simulink model "ASE_370C_MinProj2_simulink"  (R2018b)
settings: Solver=VariableStepAuto  StartTime=0.0  StopTime=20  RelTol=1e-3
InitFcn:
  | RUN_1st_ASE_370C_MiniProject1
CloseFcn:
  | ASE_370C_MiniProject1_Plots
settings Model: Creator=kenda  LastModifiedBy=kenda

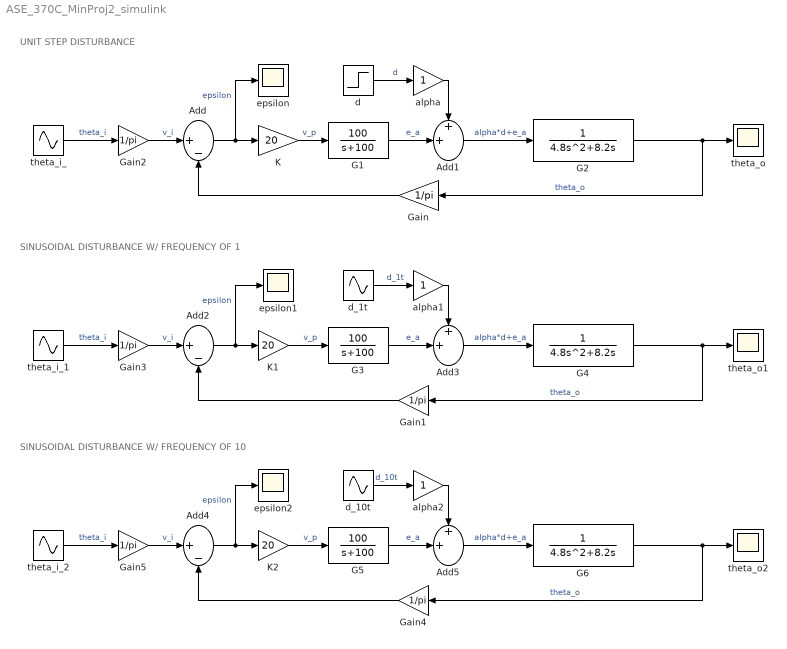
== system ASE_370C_MinProj2_simulink ==
  note: UNIT STEP DISTURBANCE
  note: SINUSOIDAL DISTURBANCE W/ FREQUENCY OF 1
  note: SINUSOIDAL DISTURBANCE W/ FREQUENCY OF 10
  Add : Sum  Inputs=|+-
  Add1 : Sum  Inputs=++|
  Add2 : Sum  Inputs=|+-
  Add3 : Sum  Inputs=++|
  Add4 : Sum  Inputs=|+-
  Add5 : Sum  Inputs=++|
  G1 : TransferFcn  Numerator=100  Denominator=[1 100]
  G2 : TransferFcn  Denominator=[4.8 8.2 0]
  G3 : TransferFcn  Numerator=100  Denominator=[1 100]
  G4 : TransferFcn  Denominator=[4.8 8.2 0]
  G5 : TransferFcn  Numerator=100  Denominator=[1 100]
  G6 : TransferFcn  Denominator=[4.8 8.2 0]
  Gain{,1..5} (6 alike) : Gain  Gain=1/pi
  K : Gain  Gain=20
  K1 : Gain  Gain=20
  K2 : Gain  Gain=20
  alpha : Gain
  alpha1 : Gain
  alpha2 : Gain
  d : Step  SampleTime=0
  d_10t : Sin  Frequency=10  SampleTime=0
  d_1t : Sin  SampleTime=0
  epsilon : Scope
  epsilon1 : Scope
  epsilon2 : Scope
  theta_i_ : Sin  Bias=1  Frequency=0  SampleTime=0
  theta_i_1 : Sin  Frequency=0  SampleTime=0
  theta_i_2 : Sin  Frequency=0  SampleTime=0
  theta_o : Scope
  theta_o1 : Scope
  theta_o2 : Scope
  wires:
  Gain2/1 -> Add/1  "v_i"
  Add/1 -> epsilon/1, K/1  "epsilon"
  K/1 -> G1/1  "v_p"
  G1/1 -> Add1/2  "e_a"
  alpha/1 -> Add1/1
  Add1/1 -> G2/1  "alpha*d+e_a"
  G2/1 -> Gain/1, theta_o/1  "theta_o"
  Gain/1 -> Add/2
  d/1 -> alpha/1  "d"
  d_1t/1 -> alpha1/1  "d_1t"
  d_10t/1 -> alpha2/1  "d_10t"
  G4/1 -> Gain1/1, theta_o1/1  "theta_o"
  Add3/1 -> G4/1  "alpha*d+e_a"
  theta_i_1/1 -> Gain3/1  "theta_i"
  Gain1/1 -> Add2/2
  Gain3/1 -> Add2/1  "v_i"
  Add2/1 -> epsilon1/1, K1/1  "epsilon"
  alpha1/1 -> Add3/1
  G3/1 -> Add3/2  "e_a"
  K1/1 -> G3/1  "v_p"
  G6/1 -> Gain4/1, theta_o2/1  "theta_o"
  Add5/1 -> G6/1  "alpha*d+e_a"
  theta_i_2/1 -> Gain5/1  "theta_i"
  Gain4/1 -> Add4/2
  Gain5/1 -> Add4/1  "v_i"
  Add4/1 -> epsilon2/1, K2/1  "epsilon"
  alpha2/1 -> Add5/1
  G5/1 -> Add5/2  "e_a"
  K2/1 -> G5/1  "v_p"
  theta_i_/1 -> Gain2/1  "theta_i"
